simulink model "MMC_MultifreqOrig"  (R2023b)
settings: Solver=ode4  StartTime=0.0  StopTime=30  FixedStep=1/(50e3)  RelTol=1e-4  EnableMultiTasking=on
settings Model: Creator=Anyalí  LastModifiedBy=anyal
settings SolverCC: AlgebraicLoopSolver=TrustRegion
settings DataIOCC: LimitDataPoints=on  SaveFormat=Array  SignalLoggingSaveFormat=ModelDataLogs  ReturnWorkspaceOutputs=off
settings OptimizationCC: ExpressionDepthLimit=2147483647  LifeSpan=inf
settings DebuggingCC: UnderspecifiedInitializationDetection=Classic  MergeDetectMultiDrivingBlocksExec=none  SolverPrmCheckMsg=warning  FcnCallInpInsideContextMsg=warning  UnconnectedInputMsg=warning  UnconnectedOutputMsg=warning  UnconnectedLineMsg=warning  AllowSymbolicDim=off  StateNameClashWarn=warning  SFUnexpectedBacktrackingDiag=warning  SFNoUnconditionalDefaultTransitionDiag=warning  SFExecutionAtInitializationDiag=none  ArithmeticOperatorsInVariantConditions=warning
settings HardwareCC: ProdBitPerPointer=32  ProdBitPerSizeT=32  ProdBitPerPtrDiffT=32  ProdLargestAtomicFloat=None  ProdIntDivRoundTo=Undefined  ProdEndianess=Unspecified  ProdWordSize=32  ProdHWDeviceType=32-bit Generic
settings ModelReferenceCC: EnableRefExpFcnMdlSchedulingChecks=on  PropagateSignalLabelsOutOfModel=off
settings SFSimCC: SimUseLocalCustomCode=off  CustomCodeUndefinedFunction=UseInterfaceOnly
settings RTWCC: RTWUseLocalCustomCode=off
settings CodeAppCC: StateflowObjectComments=on
settings GRTTargetCC: TargetLangStandard=C89/C90 (ANSI)  CombineOutputUpdateFcns=off  GRTInterface=on
settings ConfigComp: CovMetricSettings=dw  CovSaveCumulativeToWorkspaceVar=on  CovSaveSingleToWorkspaceVar=on  CovExternalEMLEnable=off
settings SimscapeCC: SimscapeNormalizeSystem=off
settings ConfigurationSet: Description=SimMechanics 2G

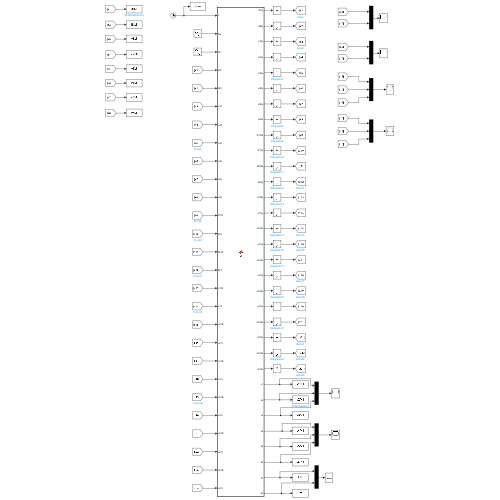
[thumbnail: Simulink's stored preview of the top-level diagram]
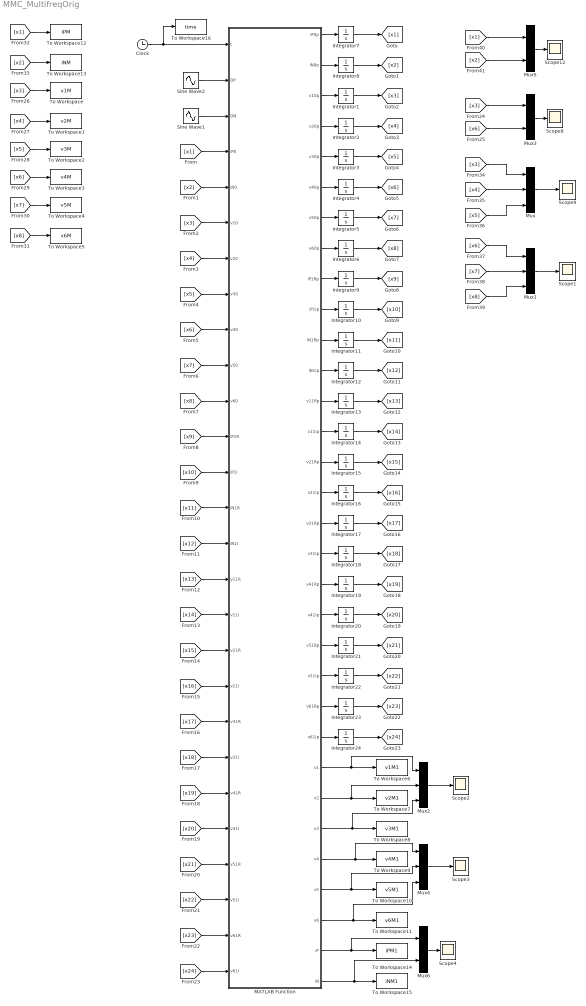
== system MMC_MultifreqOrig ==
  Clock : Clock
  Integrator1 : Integrator  InitialCondition=140
  Integrator{7..24} (18 alike) : Integrator
  Integrator2 : Integrator  InitialCondition=180
  Integrator3 : Integrator  InitialCondition=110
  Integrator4 : Integrator  InitialCondition=160
  Integrator5 : Integrator  InitialCondition=140
  Integrator6 : Integrator  InitialCondition=100
  MATLAB Function : MATLAB Function  TreatAsAtomicUnit=on
  Mux{,1..2,4} (4 alike) : Mux  Inputs=3
  Mux3 : Mux  Inputs=2
  Mux5 : Mux  Inputs=2
  Mux6 : Mux  Inputs=2
  Scope{1..4,8..9,12} (7 alike) : Scope
  Sine Wave1 : Sin  Amplitude=0.45  Bias=0.5  Frequency=100*pi  SampleTime=0
  Sine Wave2 : Sin  Amplitude=0.45  Bias=0.5  Frequency=100*pi  Phase=pi  SampleTime=0
  To Workspace : ToWorkspace  VariableName=v1M  SampleTime=-1
  To Workspace1 : ToWorkspace  VariableName=v2M  SampleTime=-1
  To Workspace10 : ToWorkspace  VariableName=v5M1  SampleTime=-1
  To Workspace11 : ToWorkspace  VariableName=v6M1  SampleTime=-1
  To Workspace12 : ToWorkspace  VariableName=iPM  SampleTime=-1
  To Workspace13 : ToWorkspace  VariableName=iNM  SampleTime=-1
  To Workspace14 : ToWorkspace  VariableName=iPM1  SampleTime=-1
  To Workspace15 : ToWorkspace  VariableName=iNM1  SampleTime=-1
  To Workspace16 : ToWorkspace  VariableName=time  SampleTime=-1
  To Workspace2 : ToWorkspace  VariableName=v3M  SampleTime=-1
  To Workspace3 : ToWorkspace  VariableName=v4M  SampleTime=-1
  To Workspace4 : ToWorkspace  VariableName=v5M  SampleTime=-1
  To Workspace5 : ToWorkspace  VariableName=v6M  SampleTime=-1
  To Workspace6 : ToWorkspace  VariableName=v1M1  SampleTime=-1
  To Workspace7 : ToWorkspace  VariableName=v2M1  SampleTime=-1
  To Workspace8 : ToWorkspace  VariableName=v3M1  SampleTime=-1
  To Workspace9 : ToWorkspace  VariableName=v4M1  SampleTime=-1
  wires:
  Sine Wave2/1 -> MATLAB Function/2(DP)
  Integrator1/1 -> [x3]
  Sine Wave1/1 -> MATLAB Function/3(DN)
  Integrator3/1 -> [x5]
  Integrator4/1 -> [x6]
  Integrator5/1 -> [x7]
  Integrator6/1 -> [x8]
  Integrator2/1 -> [x4]
  MATLAB Function/1(iP0p) -> Integrator7/1
  MATLAB Function/2(iN0p) -> Integrator8/1
  MATLAB Function/3(v10p) -> Integrator1/1
  MATLAB Function/4(v20p) -> Integrator2/1
  MATLAB Function/5(v30p) -> Integrator3/1
  MATLAB Function/6(v40p) -> Integrator4/1
  MATLAB Function/7(v50p) -> Integrator5/1
  MATLAB Function/8(v60p) -> Integrator6/1
  MATLAB Function/9(iP1Rp) -> Integrator9/1
  MATLAB Function/10(iP1Ip) -> Integrator10/1
  MATLAB Function/11(iN1Rp) -> Integrator11/1
  MATLAB Function/12(iN1Ip) -> Integrator12/1
  MATLAB Function/13(v11Rp) -> Integrator13/1
  MATLAB Function/14(v11Ip) -> Integrator14/1
  MATLAB Function/15(v21Rp) -> Integrator15/1
  MATLAB Function/16(v21Ip) -> Integrator16/1
  MATLAB Function/17(v31Rp) -> Integrator17/1
  MATLAB Function/18(v31Ip) -> Integrator18/1
  MATLAB Function/19(v41Rp) -> Integrator19/1
  MATLAB Function/20(v41Ip) -> Integrator20/1
  MATLAB Function/21(v51Rp) -> Integrator21/1
  MATLAB Function/22(v51Ip) -> Integrator22/1
  MATLAB Function/23(v61Rp) -> Integrator23/1
  MATLAB Function/24(v61Ip) -> Integrator24/1
  Integrator7/1 -> [x1]
  Integrator8/1 -> [x2]
  Integrator9/1 -> [x9]
  Integrator10/1 -> [x10]
  Integrator11/1 -> [x11]
  Integrator12/1 -> [x12]
  Integrator13/1 -> [x13]
  Integrator14/1 -> [x14]
  Integrator15/1 -> [x15]
  Integrator16/1 -> [x16]
  Integrator17/1 -> [x17]
  Integrator18/1 -> [x18]
  Integrator19/1 -> [x19]
  Integrator20/1 -> [x20]
  Integrator21/1 -> [x21]
  Integrator22/1 -> [x22]
  Integrator23/1 -> [x23]
  Integrator24/1 -> [x24]
  [x1] -> MATLAB Function/4(iP0)
  [x2] -> MATLAB Function/5(iN0)
  [x3] -> MATLAB Function/6(v10)
  [x4] -> MATLAB Function/7(v20)
  [x5] -> MATLAB Function/8(v30)
  [x6] -> MATLAB Function/9(v40)
  [x7] -> MATLAB Function/10(v50)
  [x8] -> MATLAB Function/11(v60)
  [x9] -> MATLAB Function/12(iP1R)
  [x10] -> MATLAB Function/13(iP1I)
  [x11] -> MATLAB Function/14(iN1R)
  [x12] -> MATLAB Function/15(iN1I)
  [x13] -> MATLAB Function/16(v11R)
  [x14] -> MATLAB Function/17(v11I)
  [x15] -> MATLAB Function/18(v21R)
  [x16] -> MATLAB Function/19(v21I)
  [x17] -> MATLAB Function/20(v31R)
  [x18] -> MATLAB Function/21(v31I)
  [x19] -> MATLAB Function/22(v41R)
  [x20] -> MATLAB Function/23(v41I)
  [x21] -> MATLAB Function/24(v51R)
  [x22] -> MATLAB Function/25(v51I)
  [x23] -> MATLAB Function/26(v61R)
  [x24] -> MATLAB Function/27(v61I)
  Clock/1 -> To Workspace16/1, MATLAB Function/1(t)
  [x3] -> To Workspace/1
  [x4] -> To Workspace1/1
  [x5] -> To Workspace2/1
  [x6] -> To Workspace3/1
  [x7] -> To Workspace4/1
  [x8] -> To Workspace5/1
  MATLAB Function/26(v2) -> Mux2/2, To Workspace7/1
  MATLAB Function/25(v1) -> Mux2/1, To Workspace6/1
  MATLAB Function/28(v4) -> Mux4/1, To Workspace9/1
  MATLAB Function/30(v6) -> Mux4/3, To Workspace11/1
  MATLAB Function/31(iP) -> Mux6/1, To Workspace14/1
  MATLAB Function/32(iN) -> Mux6/2, To Workspace15/1
  [x1] -> To Workspace12/1
  [x2] -> To Workspace13/1
  [x7] -> Mux1/2
  Mux1/1 -> Scope1/1
  [x6] -> Mux3/2
  [x2] -> Mux5/2
  Mux5/1 -> Scope12/1
  [x1] -> Mux5/1
  Mux/1 -> Scope9/1
  [x6] -> Mux1/1
  [x3] -> Mux3/1
  [x4] -> Mux/2
  [x3] -> Mux/1
  [x8] -> Mux1/3
  Mux3/1 -> Scope8/1
  [x5] -> Mux/3
  Mux2/1 -> Scope2/1
  MATLAB Function/27(v3) -> Mux2/3, To Workspace8/1
  Mux4/1 -> Scope3/1
  MATLAB Function/29(v5) -> Mux4/2, To Workspace10/1
  Mux6/1 -> Scope4/1

== matlab function MMC_MultifreqOrig/MATLAB Function ==
  data: t input; DP input; iP0p output; iN0p output; DN input; iP0 input; iN0 input; v10 input; v20 input; v30 input; v40 input; v10p output; v20p output; v30p output; v40p output; v50 input; v60 input; iP1R input; iP1I input; iN1R input; iN1I input; v11R input; v11I input; v21R input; v21I input; v31R input; v31I input; v41R input; v41I input; v51R input; v51I input; v61R input; v61I input; v50p output; v60p output; iP1Rp output; iP1Ip output; iN1Rp output; iN1Ip output; v11Rp output; v11Ip output; v21Rp output; v21Ip output; v31Rp output; v31Ip output; v41Rp output; v41Ip output; v51Rp output; v51Ip output; v61Rp output; v61Ip output; v1 output; v2 output; v3 output; v4 output; v5 output; v6 output; iP output; iN output
function [iP0p,iN0p,v10p,v20p,v30p,v40p,v50p,v60p,iP1Rp,iP1Ip,iN1Rp,iN1Ip,v11Rp,v11Ip,v21Rp,v21Ip,v31Rp,v31Ip,v41Rp,v41Ip,v51Rp,v51Ip,v61Rp,v61Ip,v1,v2,v3,v4,v5,v6,iP,iN] = fcn(t,DP,DN,iP0,iN0,v10,v20,v30,v40,v50,v60,iP1R,iP1I,iN1R,iN1I,v11R,v11I,v21R,v21I,v31R,v31I,v41R,v41I,v51R,v51I,v61R,v61I)
%#codegen

E=420;
C=3.2e-3;
L=1e-3;
R=16;
fc=2500;
wc=2*pi*fc;

%señales de control
u10=DP;
u20=DP;
u30=DP;
u40=DN;
u50=DN;
u60=DN;

a=pi;
%brazo superior
u11=DP*exp((0)*pi*1i)/a;
u21=DP*exp(((2/3))*pi*1i)/a;
u31=DP*exp(((4/3))*pi*1i)/a;

%brazo inferior
u41=DN*exp(0*pi*1i)/a;
u51=DN*exp((2/3)*pi*1i)/a;
u61=DN*exp((4/3)*pi*1i)/a;

u11R=real(u11);
u11I=imag(u11);

u21R=real(u21);
u21I=imag(u21);

u31R=real(u31);
u31I=imag(u31);

u41R=real(u41);
u41I=imag(u41);

u51R=real(u51);
u51I=imag(u51);

u61R=real(u61);
u61I=imag(u61);

%A1 columns
c1A1=[-R/L;R/L;u10/C;u20/C;u30/C;zeros(7,1)];
c2A1=[R/L;-R/L;0;0;0;u40/C;u50/C;u60/C;zeros(4,1)];
c3A1=[-u10/L;zeros(7,1);-u11R/L;-u11I/L;zeros(2,1)];
c4A1=[-u20/L;zeros(7,1);-u21R/L;-u21I/L;zeros(2,1)];
c5A1=[-u30/L;zeros(7,1);-u31R/L;-u31I/L;zeros(2,1)];
c6A1=[0;-u40/L;zeros(8,1);-u41R/L;-u41I/L];
c7A1=[0;-u50/L;zeros(8,1);-u51R/L;-u51I/L];
c8A1=[0;-u60/L;zeros(8,1);-u61R/L;-u61I/L];
c9A1=[0;0;2*u11R/C;2*u21R/C;2*u31R/C;0;0;0;-R/L;-wc;R/L;0];
c10A1=[0;0;2*u11I/C;2*u21I/C;2*u31I/C;0;0;0;wc;-R/L;0;R/L];
c11A1=[zeros(5,1);2*u41R/C;2*u51R/C;2*u61R/C;R/L;0;-R/L;-wc];
c12A1=[zeros(5,1);2*u41I/C;2*u51I/C;2*u61I/C;0;R/L;wc;-R/L];
A1=[c1A1 c2A1 c3A1 c4A1 c5A1 c6A1 c7A1 c8A1 c9A1 c10A1 c11A1 c12A1];

%A2 columns
c1A2=[-2*u11R/L;zeros(7,1);-u10/L;zeros(3,1)];
c2A2=[-2*u11I/L;zeros(8,1);-u10/L;0;0];
c3A2=[-2*u21R/L;zeros(7,1);-u20/L;zeros(3,1)];
c4A2=[-2*u21I/L;zeros(8,1);-u20/L;zeros(2,1)];
c5A2=[-2*u31R/L;zeros(7,1);-u30/L;zeros(3,1)];
c6A2=[-2*u31I/L;zeros(8,1);-u30/L;zeros(2,1)];
c7A2=[0;-2*u41R/L;zeros(8,1);-u40/L;0];
c8A2=[0;-2*u41I/L;zeros(9,1);-u40/L];
c9A2=[0;-2*u51R/L;zeros(8,1);-u50/L;0];
c10A2=[0;-2*u51I/L;zeros(9,1);-u50/L];
c11A2=[0;-2*u61R/L;zeros(8,1);-u60/L;0];
c12A2=[0;-2*u61I/L;zeros(9,1);-u60/L];
A2=[c1A2 c2A2 c3A2 c4A2 c5A2 c6A2 c7A2 c8A2 c9A2 c10A2 c11A2 c12A2];

%A3 columns
c1A3=[u11R/C;u11I/C;u21R/C;u21I/C;u31R/C;u31I/C;zeros(6,1)];
c2A3=[zeros(6,1);u41R/C;u41I/C;u51R/C;u51I/C;u61R/C;u61I/C];
c3A3=[zeros(12,1)];
c4A3=[zeros(12,1)];
c5A3=[zeros(12,1)];
c6A3=[zeros(12,1)];
c7A3=[zeros(12,1)];
c8A3=[zeros(12,1)];
c9A3=[u10/C;0;u20/C;0;u30/C;zeros(7,1)];
c10A3=[0;u10/C;0;u20/C;0;u30/C;zeros(6,1)];
c11A3=[zeros(6,1);u40/C;0;u50/C;0;u60/C;0];
c12A3=[zeros(7,1);u40/C;0;u50/C;0;u60/C];
A3=[c1A3 c2A3 c3A3 c4A3 c5A3 c6A3 c7A3 c8A3 c9A3 c10A3 c11A3 c12A3];

%A4 columns
c1A4=[0;-wc;zeros(10,1)];
c2A4=[wc;zeros(11,1)];
c3A4=[zeros(3,1);-wc;zeros(8,1)];
c4A4=[zeros(2,1);wc;zeros(9,1)];
c5A4=[zeros(5,1);-wc;zeros(6,1)];
c6A4=[zeros(4,1);wc;zeros(7,1)];
c7A4=[zeros(7,1);-wc;zeros(4,1)];
c8A4=[zeros(6,1);wc;zeros(5,1)];
c9A4=[zeros(9,1);-wc;0;0];
c10A4=[zeros(8,1);wc;0;0;0];
c11A4=[zeros(11,1);-wc];
c12A4=[zeros(10,1);wc;0];
A4=[c1A4 c2A4 c3A4 c4A4 c5A4 c6A4 c7A4 c8A4 c9A4 c10A4 c11A4 c12A4];

x=[iP0;iN0;v10;v20;v30;v40;v50;v60;iP1R;iP1I;iN1R;iN1I;v11R;v11I;v21R;v21I;v31R;v31I;v41R;v41I;v51R;v51I;v61R;v61I];
A=[A1 A2;A3 A4];
B=[1/(2*L);1/(2*L);zeros(22,1)];

xp=A*x+B*E;

iP0p=xp(1);
iN0p=xp(2);
v10p=xp(3);
v20p=xp(4);
v30p=xp(5);
v40p=xp(6);
v50p=xp(7);
v60p=xp(8);
iP1Rp=xp(9);
iP1Ip=xp(10);
iN1Rp=xp(11);
iN1Ip=xp(12);
v11Rp=xp(13);
v11Ip=xp(14);
v21Rp=xp(15);
v21Ip=xp(16);
v31Rp=xp(17);
v31Ip=xp(18);
v41Rp=xp(19);
v41Ip=xp(20);
v51Rp=xp(21);
v51Ip=xp(22);
v61Rp=xp(23);
v61Ip=xp(24);

v1=v10+2*(v11R*cos(wc*t)-v11I*sin(wc*t));
v2=v20+2*(v21R*cos(wc*t)-v21I*sin(wc*t));
v3=v30+2*(v31R*cos(wc*t)-v31I*sin(wc*t));

v4=v40+2*(v41R*cos(wc*t)-v41I*sin(wc*t));
v5=v50+2*(v51R*cos(wc*t)-v51I*sin(wc*t));
v6=v60+2*(v61R*cos(wc*t)-v61I*sin(wc*t));

iP=iP0+2*(iP1R*cos(wc*t)-iP1I*sin(wc*t));
iN=iN0+2*(iN1R*cos(wc*t)-iN1I*sin(wc*t));
